simulink model "velocity_tracking_decel"  (R2018b)
settings: Solver=FixedStepAuto  StartTime=0.0  StopTime=tf  FixedStep=dt  RelTol=1e-3
values from neighbouring files (symbols this model uses):
  decel = 0.2*g    (= 6.44)    [run_decel.m]
  z_delay = round(t_delay/dt)    [run_decel.m]
undefined symbols (not defined in the file or in its folder): v0
settings Model: Creator=suvo.ganguli  LastModifiedBy=suvo.ganguli

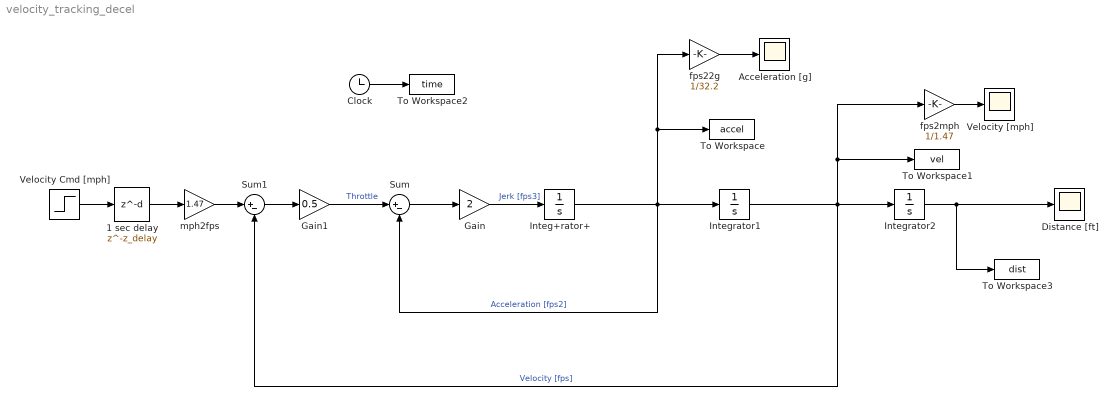
== system velocity_tracking_decel ==
  1 sec delay : Delay  DelayLength=z_delay  InitialCondition=v0
  Acceleration [g] : Scope
  Clock : Clock
  Distance [ft] : Scope
  Gain : Gain  Gain=2
  Gain1 : Gain  Gain=0.5
  Integ+rator+ : Integrator  LimitOutput=on  UpperSaturationLimit=decel  LowerSaturationLimit=-decel
  Integrator1 : Integrator  InitialCondition=v0*1.47
  Integrator2 : Integrator
  Sum : Sum  Inputs=|+-
  Sum1 : Sum  Inputs=|+-
  To Workspace : ToWorkspace  VariableName=accel  SampleTime=-1
  To Workspace1 : ToWorkspace  VariableName=vel  SampleTime=-1
  To Workspace2 : ToWorkspace  VariableName=time  SampleTime=-1
  To Workspace3 : ToWorkspace  VariableName=dist  SampleTime=-1
  Velocity [mph] : Scope
  Velocity Cmd [mph] : Step  Time=0  Before=v0  After=0  SampleTime=0
  fps22g : Gain  Gain=1/32.2
  fps2mph : Gain  Gain=1/1.47
  mph2fps : Gain  Gain=1.47
  wires:
  Sum/1 -> Gain/1
  Gain/1 -> Integ+rator+/1  "Jerk [fps3]"
  Integ+rator+/1 -> Integrator1/1, To Workspace/1, fps22g/1, Sum/2  "Acceleration [fps2]"
  Sum1/1 -> Gain1/1
  Integrator1/1 -> Sum1/2, Integrator2/1, To Workspace1/1, fps2mph/1  "Velocity [fps]"
  Gain1/1 -> Sum/1  "Throttle"
  Integrator2/1 -> To Workspace3/1, Distance [ft]/1
  fps2mph/1 -> Velocity [mph]/1
  fps22g/1 -> Acceleration [g]/1
  Clock/1 -> To Workspace2/1
  mph2fps/1 -> Sum1/1
  Velocity Cmd [mph]/1 -> 1 sec delay/1
  1 sec delay/1 -> mph2fps/1
